simulink model "ThermalControl"  (R2026b)
libraries: autolibsharedcontrolcommon x1
settings Model: Creator=The MathWorks, Inc.  LastModifiedBy=The MathWorks, Inc.

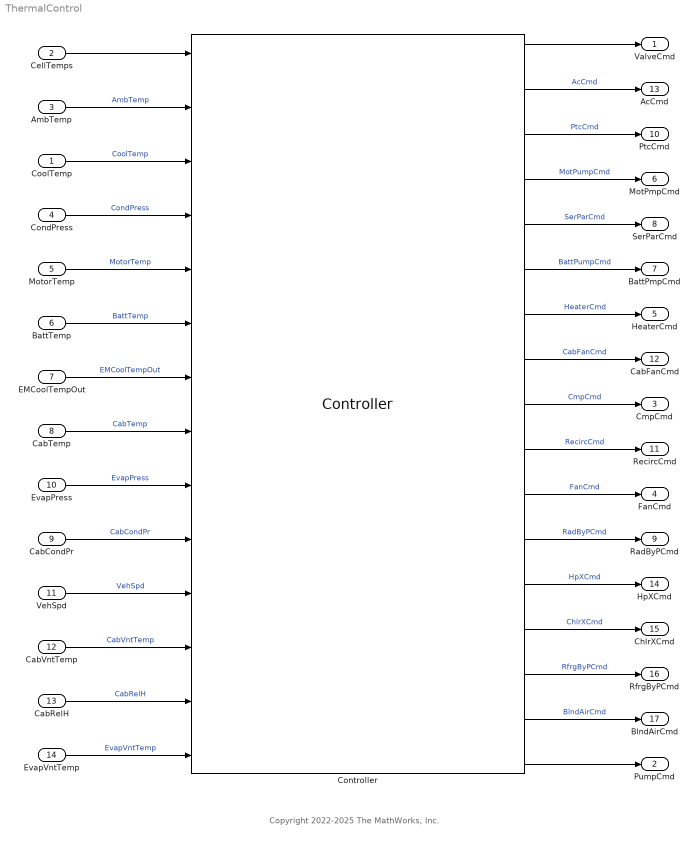
== system ThermalControl ==
  note: Copyright 2022-2025 The MathWorks, Inc.
  CoolTemp : Inport  Unit=K
  CellTemps : Inport  Port=2  PortDimensions=PlntBattNumCellSer
  AmbTemp : Inport  Port=3  Unit=K
  CondPress : Inport  Port=4  Unit=MPa
  MotorTemp : Inport  Port=5  Unit=K
  BattTemp : Inport  Port=6  Unit=K
  EMCoolTempOut : Inport  Port=7  Unit=K
  CabTemp : Inport  Port=8
  CabCondPr : Inport  Port=9
  EvapPress : Inport  Port=10
  VehSpd : Inport  Port=11
  CabVntTemp : Inport  Port=12
  CabRelH : Inport  Port=13
  EvapVntTemp : Inport  Port=14
  Controller : autolibsharedcontrolcommon/Controller  AutoState=Automatic  CabTrgT=CtrlThrCabTrgTemp  Blend=0  Recirc=0  CabFan=0  BattTrgTemp=CtrlThrBattTrgTemp  EMTrgTemp=CtrlThrEMTrgTemp  AutoON=1
  ValveCmd : Outport
  PumpCmd : Outport  Port=2
  CmpCmd : Outport  Port=3
  FanCmd : Outport  Port=4
  HeaterCmd : Outport  Port=5
  MotPmpCmd : Outport  Port=6
  BattPmpCmd : Outport  Port=7
  SerParCmd : Outport  Port=8
  RadByPCmd : Outport  Port=9
  PtcCmd : Outport  Port=10
  RecircCmd : Outport  Port=11
  CabFanCmd : Outport  Port=12
  AcCmd : Outport  Port=13
  HpXCmd : Outport  Port=14
  ChlrXCmd : Outport  Port=15
  RfrgByPCmd : Outport  Port=16
  BlndAirCmd : Outport  Port=17
  wires:
  Controller/1 -> ValveCmd/1
  CellTemps/1 -> Controller/1
  AmbTemp/1 -> Controller/2  "AmbTemp"
  CoolTemp/1 -> Controller/3  "CoolTemp"
  CondPress/1 -> Controller/4  "CondPress"
  MotorTemp/1 -> Controller/5  "MotorTemp"
  BattTemp/1 -> Controller/6  "BattTemp"
  EMCoolTempOut/1 -> Controller/7  "EMCoolTempOut"
  CabTemp/1 -> Controller/8  "CabTemp"
  EvapPress/1 -> Controller/9  "EvapPress"
  CabCondPr/1 -> Controller/10  "CabCondPr"
  VehSpd/1 -> Controller/11  "VehSpd"
  CabVntTemp/1 -> Controller/12  "CabVntTemp"
  CabRelH/1 -> Controller/13  "CabRelH"
  Controller/2 -> AcCmd/1  "AcCmd"
  Controller/3 -> PtcCmd/1  "PtcCmd"
  Controller/4 -> MotPmpCmd/1  "MotPumpCmd"
  Controller/5 -> SerParCmd/1  "SerParCmd"
  Controller/6 -> BattPmpCmd/1  "BattPumpCmd"
  Controller/7 -> HeaterCmd/1  "HeaterCmd"
  Controller/8 -> CabFanCmd/1  "CabFanCmd"
  Controller/9 -> CmpCmd/1  "CmpCmd"
  Controller/10 -> RecircCmd/1  "RecircCmd"
  Controller/11 -> FanCmd/1  "FanCmd"
  Controller/12 -> RadByPCmd/1  "RadByPCmd"
  Controller/13 -> HpXCmd/1  "HpXCmd"
  Controller/14 -> ChlrXCmd/1  "ChlrXCmd"
  Controller/15 -> RfrgByPCmd/1  "RfrgByPCmd"
  Controller/16 -> BlndAirCmd/1  "BlndAirCmd"
  EvapVntTemp/1 -> Controller/14  "EvapVntTemp"
  Controller/17 -> PumpCmd/1
